simulink model "quadcopter"  (R2024a)
settings: Solver=FixedStepAuto  StartTime=0.0  StopTime=10.0  FixedStep=0.01  RelTol=1e-3
PostLoadFcn:
  | on_model_load
StopFcn:
  | on_simulation_done
undefined symbols (not defined in the file or in its folder): ActiveScenario
libraries: csbenchlab_dist x2, csbenchlab_sys x1, csbenchlab_Controllers x1, csbenchlab_est x1, SignalEditorBlockLib x1
PostSaveFcn:
  | on_model_save
settings Model: Creator=luka  LastModifiedBy=luka

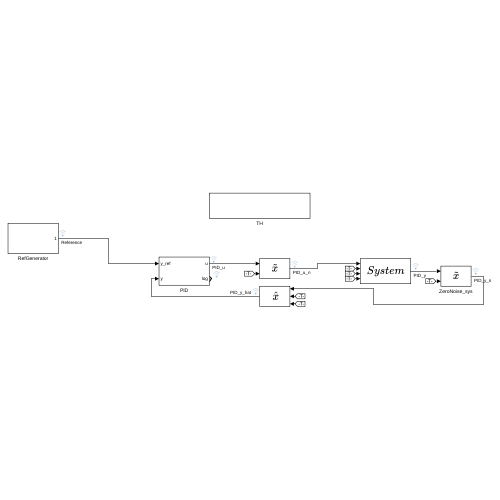
[thumbnail: Simulink's stored preview of the top-level diagram]
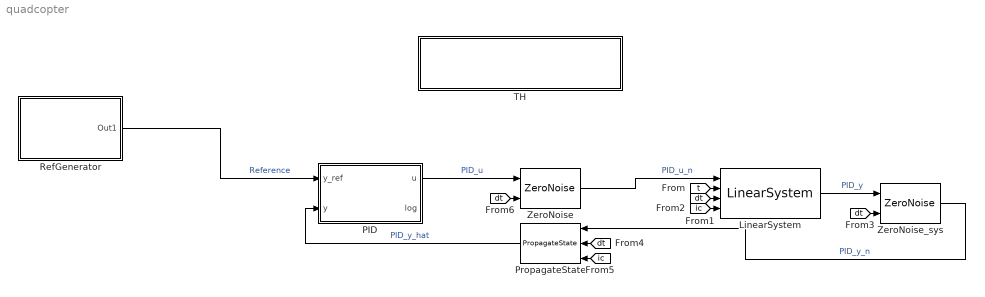
== system quadcopter ==
  LinearSystem : csbenchlab_sys/LinearSystem  Tag=__cs_m_sys;  params=CrazyFly_linearSystem  params_merged=ActiveScenario.Params  data=LinearSystem_data  ParamsType=LinearSystem_PT  DataType=LinearSystem_DT
  PID : Subsystem
  PropagateState : csbenchlab_est/PropagateState  Tag=__cs_m_est;  params=PropagateState_params  data=PropagateState_data  ParamsType=PropagateState_PT  DataType=PropagateState_DT
  RefGenerator : Subsystem  mask{scenario=P1}
      settings: OpenFcn=on_reference_generator_open();
      mask TypeOptions scenario: P1
      mask Callback scenario: on_reference_select;
      mask DialogControl edit_refs_btn Prompt: Edit references
      mask DialogControl edit_refs_btn Callback: on_edit_references_btn;
  TH : Subsystem
      mask DialogControl ParameterGroupVar Prompt: Params
  ZeroNoise : csbenchlab_dist/ZeroNoise  Tag=__cs_m_dist;  params=ZeroNoise_params  data=ZeroNoise_data  ParamsType=ZeroNoise_PT  DataType=ZeroNoise_DT
  ZeroNoise_sys : csbenchlab_dist/ZeroNoise  Tag=__cs_m_dist;  params=ZeroNoise_params  data=ZeroNoise_data  ParamsType=ZeroNoise_PT  DataType=ZeroNoise_DT
  wires:
  [t] -> LinearSystem/2
  [dt] -> LinearSystem/3
  [ic] -> LinearSystem/4
  [dt] -> ZeroNoise_sys/2
  [dt] -> PropagateState/2
  [ic] -> PropagateState/3
  [dt] -> ZeroNoise/2
  PID/1(u) -> ZeroNoise/1  "PID_u"
  ZeroNoise/1 -> LinearSystem/1  "PID_u_n"
  LinearSystem/1 -> ZeroNoise_sys/1  "PID_y"
  ZeroNoise_sys/1 -> PropagateState/1  "PID_y_n"
  PropagateState/1 -> PID/2(y)  "PID_y_hat"
  RefGenerator/1(Out1) -> PID/1(y_ref)  "Reference"

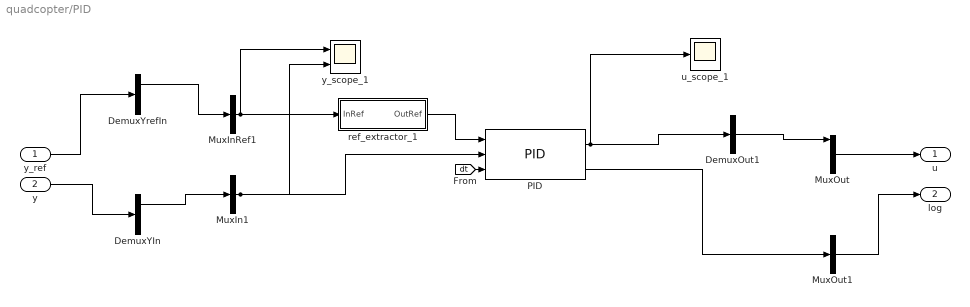
== system quadcopter/PID ==
  y_ref : Inport  PortDimensions=9
  y : Inport  Port=2  PortDimensions=9
  DemuxOut1 : Demux  Outputs=1
  DemuxYIn : Demux  Outputs=9
  DemuxYrefIn : Demux  Outputs=9
  MuxIn1 : Mux  Inputs=1
  MuxInRef1 : Mux  Inputs=1
  MuxOut : Mux
  MuxOut1 : BusCreator  Inputs=1
  PID : csbenchlab_Controllers/PID  Tag=__cs_slx_ctl;  pid_params=PID_params
  ref_extractor_1 : Subsystem
  u_scope_1 : Scope
  y_scope_1 : Scope  NumInputPorts=2
  u : Outport  PortDimensions=4
  log : Outport  Port=2
  wires:
  [dt] -> PID/3
  y/1 -> DemuxYIn/1
  y_ref/1 -> DemuxYrefIn/1
  MuxOut/1 -> u/1
  MuxOut1/1 -> log/1
  MuxInRef1/1 -> ref_extractor_1/1(InRef), y_scope_1/1
  ref_extractor_1/1(OutRef) -> PID/1
  MuxIn1/1 -> PID/2, y_scope_1/2
  PID/1 -> DemuxOut1/1, u_scope_1/1
  PID/2 -> MuxOut1/1
  DemuxYIn/3 -> MuxIn1/1
  DemuxYrefIn/3 -> MuxInRef1/1
  DemuxOut1/1 -> MuxOut/1

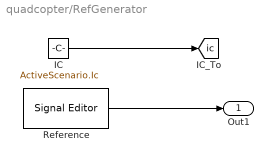
== system quadcopter/RefGenerator ==
  IC : Constant  Value=ActiveScenario.Ic
  Reference : SignalEditorBlockLib/Signal Editor  FileName=untitled.mat  ActiveScenario=Scenario  ActiveSignal=Signal 1  IsBus=off  OutputBusObjectStr=Bus: BusObject  SampleTime=0  Interpolate=off  ZeroCross=off  OutputAfterFinalValue=Setting to zero  Unit=inherit  PreserveSignalName=on  ApplySigPropsToAllScenarios=on  ApplySigPropsToAllSignals=off
  Out1 : Outport
  tag scope: ic=global
  wires:
  IC/1 -> [ic]
  Reference/1 -> Out1/1

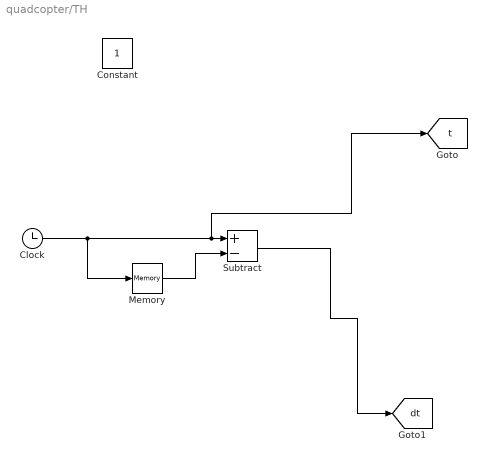
== system quadcopter/TH ==
  Clock : Clock
  Constant : Constant
  Memory : Memory
  Subtract : Sum  Inputs=+-
  tag scope: dt=global, t=global
  wires:
  Subtract/1 -> [dt]
  Memory/1 -> Subtract/2
  Clock/1 -> Memory/1, Subtract/1, [t]

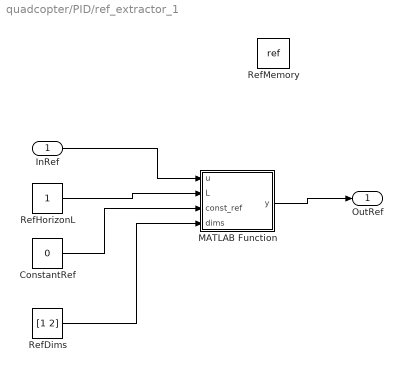
== system quadcopter/PID/ref_extractor_1 ==
  InRef : Inport
  ConstantRef : Constant  Value=0
  MATLAB Function : MATLAB Function  TreatAsAtomicUnit=on
  RefDims : Constant  Value=[1 2]
  RefHorizonL : Constant
  RefMemory : DataStoreMemory  DataStoreName=ref  WriteAfterWriteMsg=warning  ShowAdditionalParam=off  OutDataTypeStr=double
  OutRef : Outport
  wires:
  ConstantRef/1 -> MATLAB Function/3(const_ref)
  RefDims/1 -> MATLAB Function/4(dims)
  RefHorizonL/1 -> MATLAB Function/2(L)
  InRef/1 -> MATLAB Function/1(u)
  MATLAB Function/1(y) -> OutRef/1

== matlab function quadcopter/PID/ref_extractor_1/MATLAB Function ==
  settings: updateMethod=DISCRETE
  data: u input; L input; const_ref input; dims input; y output; ref data_store_memory; GlobalReference parameter
function y = fcn(u, L, const_ref, dims, GlobalReference)

persistent cnt
global ref

if isempty(cnt)
    cnt = 0;
end
cnt = cnt+1;

horizon_end = cnt+L-1;
if L > 1 
   if horizon_end > length(GlobalReference)
        if size(ref, 1) == size(u, 1)
            y = permute(ref, [2, 1]);
        else
            y = ref;
        end       
        return
   end

   if size(ref, 1) == size(u, 1)
      
      if const_ref == 0
        ref(:, :) = GlobalReference(cnt:horizon_end, dims)';
      else
        ref(:, :) = repmat(GlobalReference(cnt, dims)', 1, L);
      end
      y = permute(ref, [2, 1]);
   else
      if const_ref == 0
        ref(1:L, :) = GlobalReference(cnt:horizon_end, dims);
      else
        ref(1:L, :) = repmat(GlobalReference(cnt, dims), L, 1);
      end
      y = ref;
   end
else
   if size(ref, 1) == size(u, 1)
       ref = u;
       y = permute(ref, [2, 1]);
   else
      ref(1, :) = u';
      y = ref;
   end
end
